simulink model "PMSM_ItscSat_Model_PriusMotor_AlgebraicConst"  (R2024b)
settings: Solver=VariableStepAuto  StartTime=0.0  StopTime=0.03  FixedStep=1e-4
PostLoadFcn:
  | , if any(exist('dsrtsu_mdlpostloadfcn', 'file') == [2, 3, 6]), try dsrtsu_mdlpostloadfcn('Execute', bdroot); catch fprintf('Error in PostLoadFcn (dsrtsu_mdlpostloadfcn) for model "%s":\n %s\n', bdroot, lasterr); end, end,
undefined symbols (not defined in the file): ModelParam
libraries: simulink x1
PreSaveFcn:
  | , if any(exist('dsmpb_private', 'file') == [2, 3, 6]), try, dsmpb_private('dsmpb_mdlclblib', 'PreSave', bdroot); catch, disp(lasterr); end, end,
CloseFcn:
  | , if any(exist('dsmpb_private', 'file') == [2, 3, 6]), try, dsmpb_private('dsmpb_mdlclblib', 'Close', bdroot); catch, disp(lasterr); end, end,
settings Model: RTICANMMDATA=struct('GeneralSetupData',struct('modelroot','D:\01_XiL_SW\02_invhil-mlb_developer_3\ModuleTest','generalsettings',struct('filesettings',struct('destfolder',struct('Name','RTICANMM_FILES','Check',1),'buildfolder',struct('Name','.','Check',1),'AbsDestfolder',struct('Name','D:\01_XiL_SW\02_invhil-mlb_developer_3\ModuleTest\RTICANMM_FILES'),'AbsBuildfolder',struct('Name','D:\01_XiL_SW\02_invhil-mlb_developer_3\ModuleTest'))),'options',struct('addpaths',1,'rmpaths',1,'addtrcexclusion',logical(1),'cannavigator',struct('checkmonitoring',0),'show_usrtrc',0,'use_usrtrc',0),'advanced',struct('options',[1 1 1 1 1 1 1 1 1 1 1 1 1 1 1 1 1 1 1 1 1 1 1 1 1 1 1 1 1 1 1 1 1 1 1 1 1 1 1 1 1 1 1 1 1 1 1 1 1 1 1 1 1 1 1 1 1 1 1 1 1 1 1 1 1 1 1 1 1 1 1 1 1 1 1 1 1 1 1 1 1 1 1 1 1 1 1 1 1 1 1 1 1 1 1 1 1 1 1 1]),'MPSetup',{{}},'modelname','PMSM_Sat_Model_3ph_CrossSat_CT','block','PMSM_Sat_Model_3ph_CrossSat_CT'))  DSRTSU_INTERNAL_RTIFPGA=110  DSMPB_DATASERVER_ModelPortLibVersion1=8  DSMPB_DATASERVER_DataServerVersion1=6  DSMPB_DATASERVER_DataServerStreamVersion1=3  Creator=jkoupeny  LastModifiedBy=Tulajdonos
settings SolverCC: AlgebraicLoopSolver=TrustRegion
settings DataIOCC: ReturnWorkspaceOutputs=off
settings OptimizationCC: EfficientMapNaN2IntZero=off
settings DebuggingCC: UnconnectedInputMsg=warning  UnconnectedOutputMsg=warning  UnconnectedLineMsg=warning  ArithmeticOperatorsInVariantConditions=warning
settings HardwareCC: TargetBitPerPointer=64  TargetBitPerSizeT=64  TargetBitPerPtrDiffT=64  TargetLongLongMode=on  TargetIntDivRoundTo=Zero  TargetEndianess=LittleEndian  TargetWordSize=64  TargetHWDeviceType=MATLAB Host  ProdEqTarget=off
settings ModelReferenceCC: EnableRefExpFcnMdlSchedulingChecks=on
settings SFSimCC: SimUseLocalCustomCode=off  CustomCodeUndefinedFunction=UseInterfaceOnly
settings RTWCC: RTWUseLocalCustomCode=off  GPUComputeCapability=3.5
settings CodeAppCC: MaxIdLength=128  StateflowObjectComments=on
settings GRTTargetCC: TargetLangStandard=C89/C90 (ANSI)  CombineOutputUpdateFcns=off  GRTInterface=on

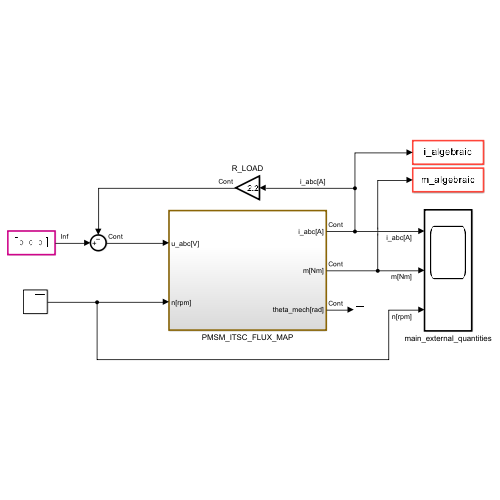
[thumbnail: Simulink's stored preview of the top-level diagram]
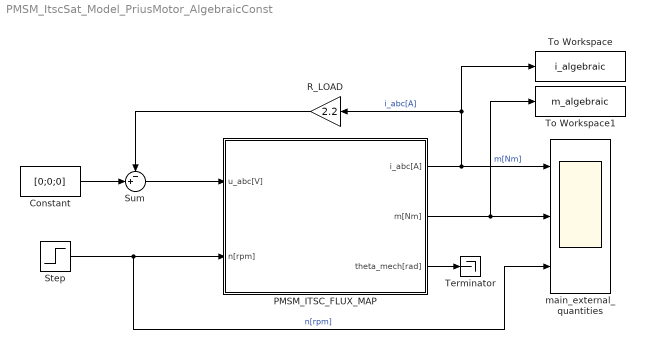
== system PMSM_ItscSat_Model_PriusMotor_AlgebraicConst ==
  Constant : Constant  Value=[0;0;0]
  PMSM_ITSC_FLUX_MAP : Subsystem
  R_LOAD : Gain  Gain=2.2
  Step : Step  Time=0  After=2500  SampleTime=0
  Sum : Sum  Inputs=-+|
  Terminator : Terminator
  To Workspace : ToWorkspace  VariableName=i_algebraic  SaveFormat=Timeseries  SampleTime=1e-4
  To Workspace1 : ToWorkspace  VariableName=m_algebraic  SaveFormat=Timeseries  SampleTime=1e-4
  main_external_quantities : Scope  NumInputPorts=3
  wires:
  PMSM_ITSC_FLUX_MAP/2(m[Nm]) -> main_external_quantities/2, To Workspace1/1  "m[Nm]"
  Step/1 -> PMSM_ITSC_FLUX_MAP/2(n[rpm]), main_external_quantities/3  "n[rpm]"
  PMSM_ITSC_FLUX_MAP/1(i_abc[A]) -> To Workspace/1, R_LOAD/1, main_external_quantities/1  "i_abc[A]"
  Sum/1 -> PMSM_ITSC_FLUX_MAP/1(u_abc[V])
  Constant/1 -> Sum/2
  R_LOAD/1 -> Sum/1
  PMSM_ITSC_FLUX_MAP/3(theta_mech[rad]) -> Terminator/1

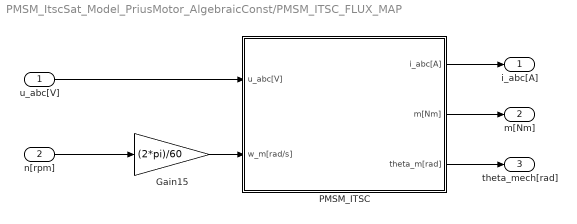
== system PMSM_ItscSat_Model_PriusMotor_AlgebraicConst/PMSM_ITSC_FLUX_MAP ==
  u_abc[V] : Inport
  n[rpm] : Inport  Port=2
  Gain15 : Gain  Gain=(2*pi)/60
  PMSM_ITSC : Subsystem
  i_abc[A] : Outport
  m[Nm] : Outport  Port=2
  theta_mech[rad] : Outport  Port=3
  wires:
  n[rpm]/1 -> Gain15/1
  Gain15/1 -> PMSM_ITSC/2(w_m[rad/s])
  PMSM_ITSC/2(m[Nm]) -> m[Nm]/1
  PMSM_ITSC/3(theta_m[rad]) -> theta_mech[rad]/1
  PMSM_ITSC/1(i_abc[A]) -> i_abc[A]/1
  u_abc[V]/1 -> PMSM_ITSC/1(u_abc[V])

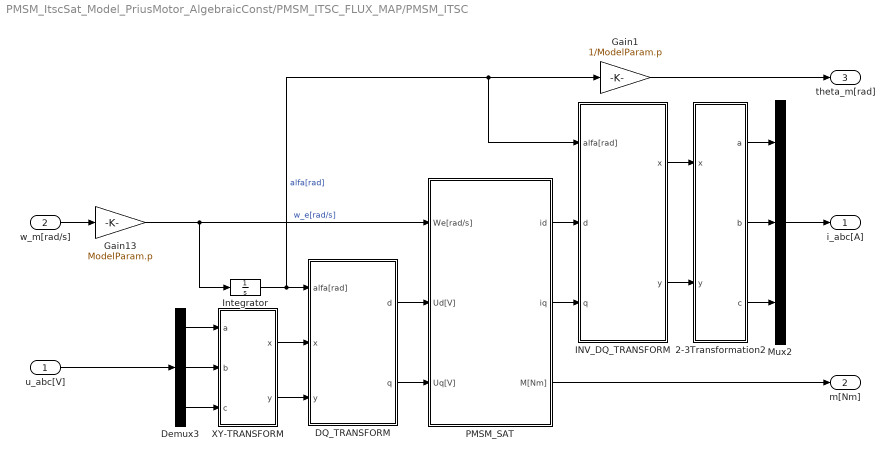
== system PMSM_ItscSat_Model_PriusMotor_AlgebraicConst/PMSM_ITSC_FLUX_MAP/PMSM_ITSC ==
  u_abc[V] : Inport
  w_m[rad/s] : Inport  Port=2
  2-3Transformation2 : Subsystem
  DQ_TRANSFORM : Subsystem
  Demux3 : Demux  Outputs=3
  Gain1 : Gain  Gain=1/ModelParam.p
  Gain13 : Gain  Gain=ModelParam.p
  INV_DQ_TRANSFORM : Subsystem
  Integrator : Integrator
  Mux2 : Mux  Inputs=3
  PMSM_SAT : Subsystem
  XY-TRANSFORM : Subsystem
  i_abc[A] : Outport
  m[Nm] : Outport  Port=2
  theta_m[rad] : Outport  Port=3
  wires:
  2-3Transformation2/1(a) -> Mux2/1
  Gain1/1 -> theta_m[rad]/1
  w_m[rad/s]/1 -> Gain13/1
  Gain13/1 -> Integrator/1, PMSM_SAT/1(We[rad/s])  "w_e[rad/s]"
  u_abc[V]/1 -> Demux3/1
  XY-TRANSFORM/2(y) -> DQ_TRANSFORM/3(y)
  XY-TRANSFORM/1(x) -> DQ_TRANSFORM/2(x)
  DQ_TRANSFORM/2(q) -> PMSM_SAT/3(Uq[V])
  DQ_TRANSFORM/1(d) -> PMSM_SAT/2(Ud[V])
  Demux3/2 -> XY-TRANSFORM/2(b)
  Demux3/1 -> XY-TRANSFORM/1(a)
  Demux3/3 -> XY-TRANSFORM/3(c)
  PMSM_SAT/2(iq) -> INV_DQ_TRANSFORM/3(q)
  PMSM_SAT/1(id) -> INV_DQ_TRANSFORM/2(d)
  Integrator/1 -> INV_DQ_TRANSFORM/1(alfa[rad]), Gain1/1, DQ_TRANSFORM/1(alfa[rad])  "alfa[rad]"
  INV_DQ_TRANSFORM/2(y) -> 2-3Transformation2/2(y)
  INV_DQ_TRANSFORM/1(x) -> 2-3Transformation2/1(x)
  Mux2/1 -> i_abc[A]/1
  2-3Transformation2/2(b) -> Mux2/2
  2-3Transformation2/3(c) -> Mux2/3
  PMSM_SAT/3(M[Nm]) -> m[Nm]/1

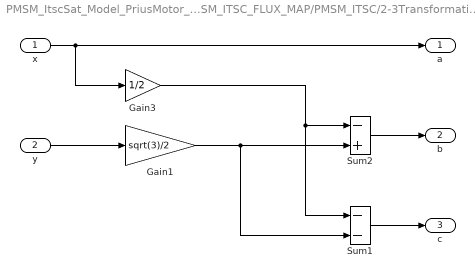
== system PMSM_ItscSat_Model_PriusMotor_AlgebraicConst/PMSM_ITSC_FLUX_MAP/PMSM_ITSC/2-3Transformation2 ==
  x : Inport
  y : Inport  Port=2
  Gain1 : Gain  Gain=sqrt(3)/2  SaturateOnIntegerOverflow=on  OutDataTypeStr=Inherit: Same as input  ParamDataTypeStr=Inherit: Same as input
  Gain3 : Gain  Gain=1/2  SaturateOnIntegerOverflow=on  OutDataTypeStr=Inherit: Same as input  ParamDataTypeStr=Inherit: Same as input
  Sum1 : Sum  Inputs=--  InputSameDT=on  SaturateOnIntegerOverflow=on  OutDataTypeStr=Inherit: Same as first input
  Sum2 : Sum  Inputs=-+  InputSameDT=on  SaturateOnIntegerOverflow=on  OutDataTypeStr=Inherit: Same as first input
  a : Outport
  b : Outport  Port=2
  c : Outport  Port=3
  wires:
  Gain3/1 -> Sum2/1, Sum1/1
  Gain1/1 -> Sum1/2, Sum2/2
  x/1 -> Gain3/1, a/1
  Sum1/1 -> c/1
  y/1 -> Gain1/1
  Sum2/1 -> b/1

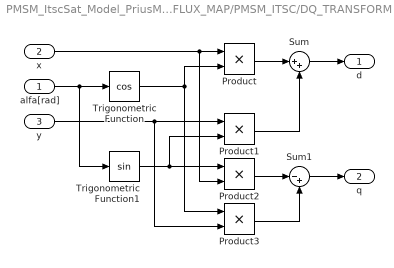
== system PMSM_ItscSat_Model_PriusMotor_AlgebraicConst/PMSM_ITSC_FLUX_MAP/PMSM_ITSC/DQ_TRANSFORM ==
  alfa[rad] : Inport
  x : Inport  Port=2
  y : Inport  Port=3
  Product{,1..3} (4 alike) : Product  RndMeth=Zero
  Sum : Sum  Inputs=|++
  Sum1 : Sum  Inputs=|-+
  Trigonometric Function : Trigonometry  Operator=cos
  Trigonometric Function1 : Trigonometry
  d : Outport
  q : Outport  Port=2
  wires:
  x/1 -> Product/1, Product2/2
  alfa[rad]/1 -> Trigonometric Function/1, Trigonometric Function1/1
  Product/1 -> Sum/1
  Product1/1 -> Sum/2
  Sum/1 -> d/1
  Trigonometric Function/1 -> Product/2, Product3/1
  y/1 -> Product1/1, Product3/2
  Trigonometric Function1/1 -> Product1/2, Product2/1
  Product2/1 -> Sum1/1
  Product3/1 -> Sum1/2
  Sum1/1 -> q/1

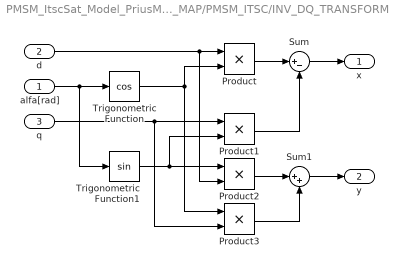
== system PMSM_ItscSat_Model_PriusMotor_AlgebraicConst/PMSM_ITSC_FLUX_MAP/PMSM_ITSC/INV_DQ_TRANSFORM ==
  alfa[rad] : Inport
  d : Inport  Port=2
  q : Inport  Port=3
  Product{,1..3} (4 alike) : Product  RndMeth=Zero
  Sum : Sum  Inputs=|+-
  Sum1 : Sum  Inputs=|++
  Trigonometric Function : Trigonometry  Operator=cos
  Trigonometric Function1 : Trigonometry
  x : Outport
  y : Outport  Port=2
  wires:
  Sum1/1 -> y/1
  Product3/1 -> Sum1/2
  Product2/1 -> Sum1/1
  Trigonometric Function1/1 -> Product2/1, Product1/2
  q/1 -> Product3/2, Product1/1
  Trigonometric Function/1 -> Product3/1, Product/2
  Sum/1 -> x/1
  Product1/1 -> Sum/2
  Product/1 -> Sum/1
  alfa[rad]/1 -> Trigonometric Function1/1, Trigonometric Function/1
  d/1 -> Product2/2, Product/1

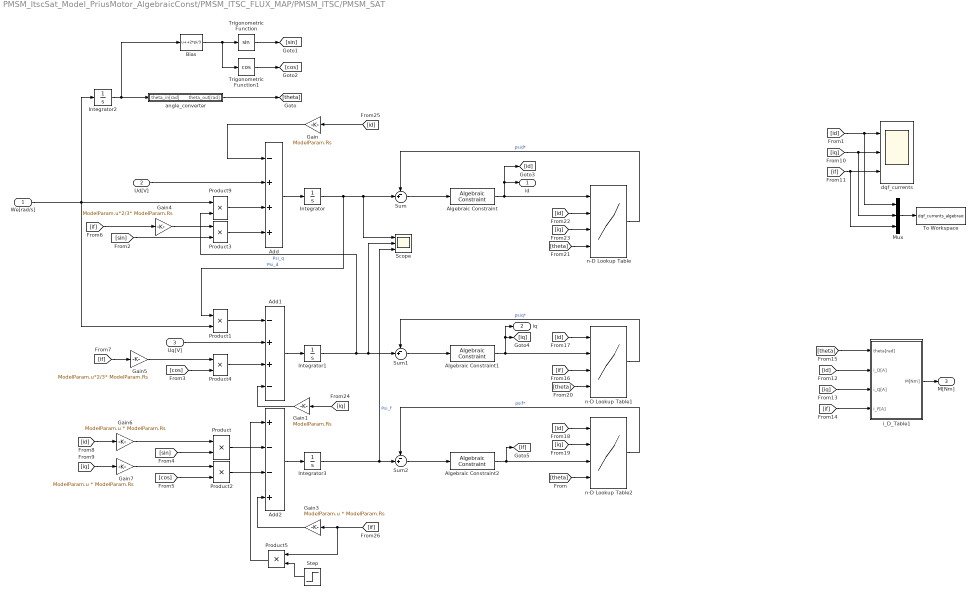
== system PMSM_ItscSat_Model_PriusMotor_AlgebraicConst/PMSM_ITSC_FLUX_MAP/PMSM_ITSC/PMSM_SAT ==
  We[rad/s] : Inport
  Ud[V] : Inport  Port=2
  Uq[V] : Inport  Port=3
  Add : Sum  Inputs=-+++
  Add1 : Sum  Inputs=-++-
  Add2 : Sum  Inputs=+--+
  Algebraic Constraint : AlgebraicConstraint
  Algebraic Constraint1 : AlgebraicConstraint
  Algebraic Constraint2 : AlgebraicConstraint
  Bias : Bias  Bias=+2*pi/3  SaturateOnIntegerOverflow=off
  Gain : Gain  Gain=ModelParam.Rs
  Gain1 : Gain  Gain=ModelParam.Rs
  Gain3 : Gain  Gain=ModelParam.u * ModelParam.Rs
  Gain4 : Gain  Gain=ModelParam.u*2/3* ModelParam.Rs
  Gain5 : Gain  Gain=ModelParam.u*2/3* ModelParam.Rs
  Gain6 : Gain  Gain=ModelParam.u * ModelParam.Rs
  Gain7 : Gain  Gain=ModelParam.u * ModelParam.Rs
  Integrator : Integrator  InitialCondition=ModelParam.MachineModel.PsidInit
  Integrator1 : Integrator  InitialCondition=ModelParam.MachineModel.PsiqInit
  Integrator2 : Integrator
  Integrator3 : Integrator  InitialCondition=ModelParam.MachineModel.PsifInit
  Mux : Mux  Inputs=3
  Product : Product
  Product{1,3..4,9} (4 alike) : Product  RndMeth=Zero
  Product2 : Product
  Product5 : Product
  Scope : Scope  NumInputPorts=3
  Step : Step  Time=0.015  Before=ModelParam.Rf  After=ModelParam.Rf/10  SampleTime=0
  Sum : Sum  Inputs=-+|
  Sum1 : Sum  Inputs=-+|
  Sum2 : Sum  Inputs=-+|
  To Workspace : ToWorkspace  VariableName=dqf_currents_algebraic  SaveFormat=Timeseries  SampleTime=1e-4
  Trigonometric Function : Trigonometry
  Trigonometric Function1 : Trigonometry  Operator=cos
  angle_converter : Subsystem
  dqf_currents : Scope  NumInputPorts=3
  i_D_Table1 : Subsystem
  n-D Lookup Table : Lookup_n-D  NumberOfTableDimensions=4  BreakpointsForDimension1=ModelParam.MachineModel.IdGrid  BreakpointsForDimension2=ModelParam.MachineModel.IqGrid  BreakpointsForDimension3=ModelParam.MachineModel.IfGrid  BreakpointsForDimension4=ModelParam.MachineModel.ThetaGrid  Table=ModelParam.MachineModel.PsidMap  InternalRulePriority=Speed  RndMeth=Simplest
      settings: InputPortMap=u0,u1,u2,u3
  n-D Lookup Table1 : Lookup_n-D  NumberOfTableDimensions=4  BreakpointsForDimension1=ModelParam.MachineModel.IdGrid  BreakpointsForDimension2=ModelParam.MachineModel.IqGrid  BreakpointsForDimension3=ModelParam.MachineModel.IfGrid  BreakpointsForDimension4=ModelParam.MachineModel.ThetaGrid  Table=ModelParam.MachineModel.PsiqMap  InternalRulePriority=Speed  RndMeth=Simplest
      settings: InputPortMap=u0,u1,u2,u3
  n-D Lookup Table2 : Lookup_n-D  NumberOfTableDimensions=4  BreakpointsForDimension1=ModelParam.MachineModel.IdGrid  BreakpointsForDimension2=ModelParam.MachineModel.IqGrid  BreakpointsForDimension3=ModelParam.MachineModel.IfGrid  BreakpointsForDimension4=ModelParam.MachineModel.ThetaGrid  Table=ModelParam.MachineModel.PsifMap  InternalRulePriority=Speed  RndMeth=Simplest
      settings: InputPortMap=u0,u1,u2,u3
  id : Outport
  iq : Outport  Port=2
  M[Nm] : Outport  Port=3
  wires:
  Add1/1 -> Integrator1/1
  Uq[V]/1 -> Add1/2
  Ud[V]/1 -> Add/2
  Add/1 -> Integrator/1
  We[rad/s]/1 -> Product1/2, Integrator2/1, Product9/1
  Integrator/1 -> Scope/1, Sum/2, Product1/1  "Psi_d"
  Integrator1/1 -> Scope/2, Sum1/2, Product9/2  "Psi_q"
  Gain/1 -> Add/1
  Gain1/1 -> Add1/4
  i_D_Table1/1(M[Nm]) -> M[Nm]/1
  Product9/1 -> Add/3
  Product1/1 -> Add1/1
  Add2/1 -> Integrator3/1
  angle_converter/1(theta_out[rad]) -> [theta]
  Integrator2/1 -> Bias/1, angle_converter/1(theta_in[rad])
  Trigonometric Function/1 -> [sin]
  Trigonometric Function1/1 -> [cos]
  Product/1 -> Add2/2
  Product2/1 -> Add2/3
  [sin] -> Product/2
  [cos] -> Product2/2
  Product5/1 -> Add2/1
  Gain3/1 -> Add2/4
  [if] -> Gain4/1
  Product3/1 -> Add/4
  Gain4/1 -> Product3/1
  [sin] -> Product3/2
  Product4/1 -> Add1/3
  [if] -> Gain5/1
  Gain5/1 -> Product4/1
  [cos] -> Product4/2
  [id] -> Gain6/1
  [iq] -> Gain7/1
  Gain7/1 -> Product2/1
  Gain6/1 -> Product/1
  Bias/1 -> Trigonometric Function1/1, Trigonometric Function/1
  Step/1 -> Product5/2
  [id] -> i_D_Table1/2(i_D[A])
  [iq] -> i_D_Table1/3(i_Q[A])
  [if] -> i_D_Table1/4(i_F[A])
  [theta] -> i_D_Table1/1(theta[rad])
  Integrator3/1 -> Scope/3, Sum2/2  "Psi_f"
  Sum/1 -> Algebraic Constraint/1
  Sum1/1 -> Algebraic Constraint1/1
  Sum2/1 -> Algebraic Constraint2/1
  n-D Lookup Table/1 -> Sum/1  "psid*"
  Algebraic Constraint/1 -> [id], id/1, n-D Lookup Table/1
  Algebraic Constraint1/1 -> n-D Lookup Table1/2, iq/1, [iq]
  Algebraic Constraint2/1 -> n-D Lookup Table2/3, [if]
  n-D Lookup Table1/1 -> Sum1/1  "psiq*"
  n-D Lookup Table2/1 -> Sum2/1  "psif*"
  [theta] -> n-D Lookup Table2/4
  [if] -> n-D Lookup Table1/3
  [id] -> n-D Lookup Table1/1
  [id] -> n-D Lookup Table2/1
  [iq] -> n-D Lookup Table2/2
  [theta] -> n-D Lookup Table1/4
  [theta] -> n-D Lookup Table/4
  [id] -> n-D Lookup Table/2
  [iq] -> n-D Lookup Table/3
  [iq] -> Gain1/1
  [id] -> Gain/1
  [if] -> Product5/1, Gain3/1
  Mux/1 -> To Workspace/1
  [id] -> Mux/1, dqf_currents/1
  [iq] -> Mux/2, dqf_currents/2
  [if] -> Mux/3, dqf_currents/3

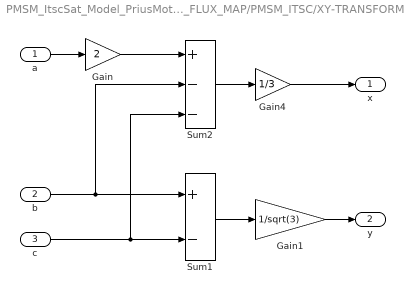
== system PMSM_ItscSat_Model_PriusMotor_AlgebraicConst/PMSM_ITSC_FLUX_MAP/PMSM_ITSC/XY-TRANSFORM ==
  a : Inport
  b : Inport  Port=2
  c : Inport  Port=3
  Gain : Gain  Gain=2  SaturateOnIntegerOverflow=on  OutDataTypeStr=Inherit: Same as input  ParamDataTypeStr=Inherit: Same as input
  Gain1 : Gain  Gain=1/sqrt(3)  SaturateOnIntegerOverflow=on  OutDataTypeStr=Inherit: Same as input  ParamDataTypeStr=Inherit: Same as input
  Gain4 : Gain  Gain=1/3  SaturateOnIntegerOverflow=on  OutDataTypeStr=Inherit: Same as input  ParamDataTypeStr=Inherit: Same as input
  Sum1 : Sum  Inputs=+-  InputSameDT=on  SaturateOnIntegerOverflow=on  OutDataTypeStr=Inherit: Same as first input
  Sum2 : Sum  Inputs=+--  InputSameDT=on  SaturateOnIntegerOverflow=on  OutDataTypeStr=Inherit: Same as first input
  x : Outport
  y : Outport  Port=2
  wires:
  a/1 -> Gain/1
  Sum1/1 -> Gain1/1
  Gain1/1 -> y/1
  b/1 -> Sum1/1, Sum2/2
  c/1 -> Sum1/2, Sum2/3
  Gain/1 -> Sum2/1
  Sum2/1 -> Gain4/1
  Gain4/1 -> x/1

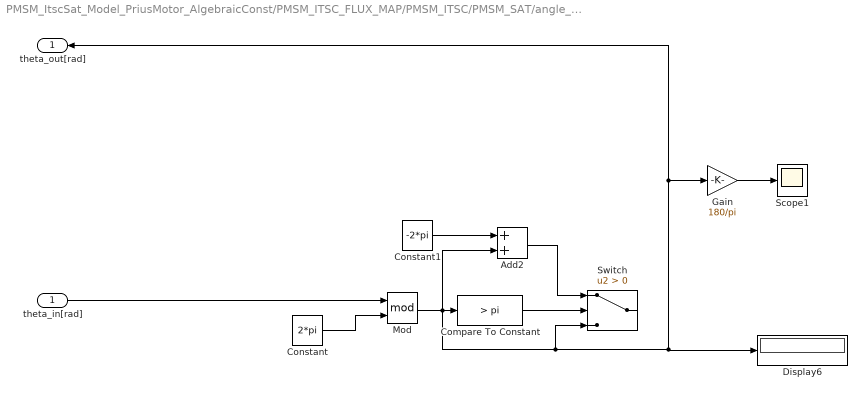
== system PMSM_ItscSat_Model_PriusMotor_AlgebraicConst/PMSM_ITSC_FLUX_MAP/PMSM_ITSC/PMSM_SAT/angle_converter ==
  theta_in[rad] : Inport
  Add2 : Sum
  Compare To Constant : simulink/Logic and Bit Operations/Compare To Constant  relop=>  const=pi  OutDataTypeStr=boolean  ZeroCross=off
  Constant : Constant  Value=2*pi
  Constant1 : Constant  Value=-2*pi
  Display6 : Display
  Gain : Gain  Gain=180/pi
  Mod : Math  Operator=mod
  Scope1 : Scope
  Switch : Switch  Criteria=u2 > Threshold  SaturateOnIntegerOverflow=off  InputSameDT=off
  theta_out[rad] : Outport
  wires:
  Mod/1 -> Add2/2, Display6/1, theta_out[rad]/1, Gain/1, Switch/3, Compare To Constant/1
  Constant1/1 -> Add2/1
  Constant/1 -> Mod/2
  Compare To Constant/1 -> Switch/2
  Add2/1 -> Switch/1
  theta_in[rad]/1 -> Mod/1
  Gain/1 -> Scope1/1

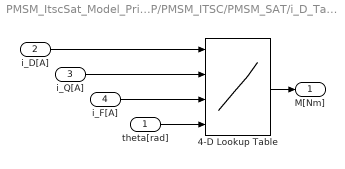
== system PMSM_ItscSat_Model_PriusMotor_AlgebraicConst/PMSM_ITSC_FLUX_MAP/PMSM_ITSC/PMSM_SAT/i_D_Table1 ==
  theta[rad] : Inport
  i_D[A] : Inport  Port=2
  i_Q[A] : Inport  Port=3
  i_F[A] : Inport  Port=4
  4-D Lookup Table : Lookup_n-D  NumberOfTableDimensions=4  BreakpointsForDimension1=ModelParam.MachineModel.IdGrid  BreakpointsForDimension2=ModelParam.MachineModel.IqGrid  BreakpointsForDimension3=ModelParam.MachineModel.IfGrid  BreakpointsForDimension4=ModelParam.MachineModel.ThetaGrid  Table=ModelParam.MachineModel.TorqueMap  InterpMethod=Cubic spline  InternalRulePriority=Speed  RndMeth=Simplest
      settings: InputPortMap=u0,u1,u2,u3
  M[Nm] : Outport
  wires:
  i_F[A]/1 -> 4-D Lookup Table/3
  theta[rad]/1 -> 4-D Lookup Table/4
  4-D Lookup Table/1 -> M[Nm]/1
  i_Q[A]/1 -> 4-D Lookup Table/2
  i_D[A]/1 -> 4-D Lookup Table/1
